simulink model "ParameterTest_LQR"  (R2018b)
settings: Solver=VariableStepAuto  StartTime=0.0  StopTime=10.0  RelTol=1e-3
settings Model: Creator=danial  LastModifiedBy=danial

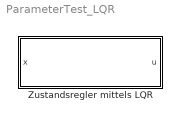
== system ParameterTest_LQR ==
  Zustandsregler mittels LQR : MATLAB Function  TreatAsAtomicUnit=on

== matlab function ParameterTest_LQR/Zustandsregler mittels LQR ==
  data: u output; x input
function u = Zustandsregler_LQR(x) %#codegen

%% Implementierung des Zustandsreglers mit LQR
K =[-0.4099,   -2.1232,   -3.4807,   -0.3483];
u = -K*x;
